simulink model "AAIver2"  (R2022a)
settings: Solver=FixedStepAuto  StartTime=0.0  StopTime=10.0  FixedStep=1e-3  RelTol=1e-3  EnableMultiTasking=on
undefined symbols (not defined in the file): D0, D10, D11, D13, D2, D3, D4, D5, D8, D9, PTA0, PTA1, PTA2, PTB23, PTB9, PTC16, PTC4, PTD0, PTD1, PTD2
libraries: frdmk64flib x10
settings Model: ExtModeTrigDuration=5  Creator=bmile  LastModifiedBy=Motz
settings OptimizationCC: EnhancedBackFolding=on  PassReuseOutputArgsAs=Individual arguments  ZeroExternalMemoryAtStartup=off  ZeroInternalMemoryAtStartup=off  MaxStackSize=64  OptimizeBlockOrder=speed  DifferentSizesBufferReuse=on  OptimizationCustomize=off  EfficientTunableParamExpr=on
settings DebuggingCC: ParameterTunabilityLossMsg=error
settings HardwareCC: ProdBitPerPointer=32  ProdBitPerSizeT=32  ProdBitPerPtrDiffT=32  ProdLargestAtomicInteger=Long  ProdLargestAtomicFloat=Double  ProdWordSize=32  ProdHWDeviceType=ARM Compatible->ARM Cortex
settings SFSimCC: MATLABDynamicMemAlloc=off
settings RTWCC: SystemTargetFile=ert.tlc  HardwareBoard=NXP FRDM-K64F  TLCOptions="-aInlineSetEventsForThisBaseRateFcn=TLC_FALSE -aSuppressMultiTaskScheduler=TLC_FALSE  -aRateBasedStepFcn=0"  TemplateMakefile=ert_default_tmf  Toolchain=GNU Tools for ARM Embedded Processors
settings CodeAppCC: ForceParamTrailComments=on  IgnoreCustomStorageClasses=off  OperatorAnnotations=on  SimulinkDataObjDesc=on  SFDataObjDesc=on  InsertBlockDesc=on
settings ERTTargetCC: ExtModeTransport=4  ExtModeMexFile=sendToCommService

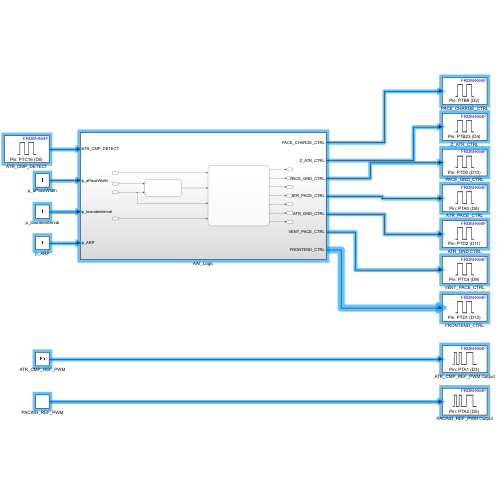
[thumbnail: Simulink's stored preview of the top-level diagram]
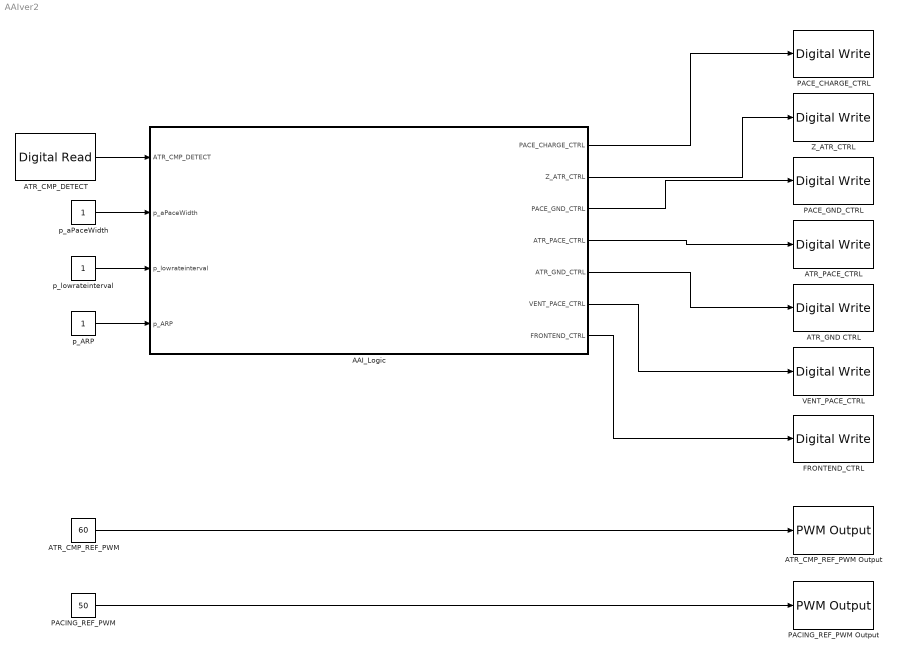
== system AAIver2 ==
  AAI_Logic : Subsystem
  ATR_CMP_DETECT : frdmk64flib/Digital Read  Whichpin=PTC16 (D0)  SampleTime=-1
  ATR_CMP_REF_PWM : Constant  Value=60
  ATR_CMP_REF_PWM Output : frdmk64flib/PWM Output  Whichpin=PTA1 (D3)  InitialFrequency=2000  InitialDutyCycle=0
  ATR_GND CTRL : frdmk64flib/Digital Write  Whichpin=PTD2 (D11)
  ATR_PACE_CTRL : frdmk64flib/Digital Write  Whichpin=PTA0 (D8)
  FRONTEND_CTRL : frdmk64flib/Digital Write  Whichpin=PTD1 (D13)
  PACE_CHARGE_CTRL : frdmk64flib/Digital Write  Whichpin=PTB9 (D2)
  PACE_GND_CTRL : frdmk64flib/Digital Write  Whichpin=PTD0 (D10)
  PACING_REF_PWM : Constant  Value=50
  PACING_REF_PWM Output : frdmk64flib/PWM Output  Whichpin=PTA2 (D5)  InitialFrequency=2000  InitialDutyCycle=0
  VENT_PACE_CTRL : frdmk64flib/Digital Write  Whichpin=PTC4 (D9)
  Z_ATR_CTRL : frdmk64flib/Digital Write  Whichpin=PTB23 (D4)
  p_ARP : Constant
  p_aPaceWidth : Constant
  p_lowrateinterval : Constant
  wires:
  PACING_REF_PWM/1 -> PACING_REF_PWM Output/1
  AAI_Logic/3(PACE_GND_CTRL) -> PACE_GND_CTRL/1
  AAI_Logic/2(Z_ATR_CTRL) -> Z_ATR_CTRL/1
  AAI_Logic/5(ATR_GND_CTRL) -> ATR_GND CTRL/1
  AAI_Logic/4(ATR_PACE_CTRL) -> ATR_PACE_CTRL/1
  p_ARP/1 -> AAI_Logic/4(p_ARP)
  p_lowrateinterval/1 -> AAI_Logic/3(p_lowrateinterval)
  AAI_Logic/6(VENT_PACE_CTRL) -> VENT_PACE_CTRL/1
  ATR_CMP_DETECT/1 -> AAI_Logic/1(ATR_CMP_DETECT)
  p_aPaceWidth/1 -> AAI_Logic/2(p_aPaceWidth)
  ATR_CMP_REF_PWM/1 -> ATR_CMP_REF_PWM Output/1
  AAI_Logic/1(PACE_CHARGE_CTRL) -> PACE_CHARGE_CTRL/1
  AAI_Logic/7(FRONTEND_CTRL) -> FRONTEND_CTRL/1

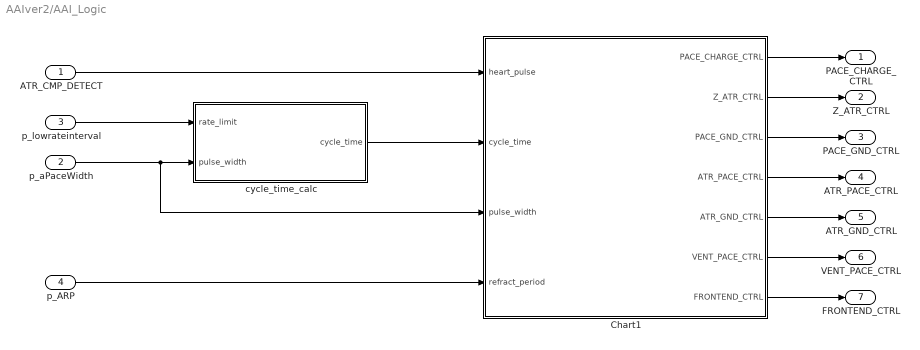
== system AAIver2/AAI_Logic ==
  ATR_CMP_DETECT : Inport
  p_aPaceWidth : Inport  Port=2
  p_lowrateinterval : Inport  Port=3
  p_ARP : Inport  Port=4
  Chart1 : Stateflow chart  TreatAsAtomicUnit=on
  cycle_time_calc : Stateflow chart  TreatAsAtomicUnit=on
  PACE_CHARGE_CTRL : Outport
  Z_ATR_CTRL : Outport  Port=2
  PACE_GND_CTRL : Outport  Port=3
  ATR_PACE_CTRL : Outport  Port=4
  ATR_GND_CTRL : Outport  Port=5
  VENT_PACE_CTRL : Outport  Port=6
  FRONTEND_CTRL : Outport  Port=7
  wires:
  cycle_time_calc/1(cycle_time) -> Chart1/2(cycle_time)
  Chart1/7(FRONTEND_CTRL) -> FRONTEND_CTRL/1
  Chart1/6(VENT_PACE_CTRL) -> VENT_PACE_CTRL/1
  Chart1/5(ATR_GND_CTRL) -> ATR_GND_CTRL/1
  Chart1/4(ATR_PACE_CTRL) -> ATR_PACE_CTRL/1
  Chart1/3(PACE_GND_CTRL) -> PACE_GND_CTRL/1
  Chart1/2(Z_ATR_CTRL) -> Z_ATR_CTRL/1
  Chart1/1(PACE_CHARGE_CTRL) -> PACE_CHARGE_CTRL/1
  p_ARP/1 -> Chart1/4(refract_period)
  p_aPaceWidth/1 -> Chart1/3(pulse_width), cycle_time_calc/2(pulse_width)
  p_lowrateinterval/1 -> cycle_time_calc/1(rate_limit)
  ATR_CMP_DETECT/1 -> Chart1/1(heart_pulse)

== stateflow chart AAIver2/AAI_Logic/cycle_time_calc ==
  state Calc_time
    entry:
    cycle_time=((1/rate_limit)*60000)-pulse_width
  (default) -> (junction 19)
  (junction 19) -> Calc_time
  data: rate_limit input; cycle_time output; pulse_width input

== stateflow chart AAIver2/AAI_Logic/Chart1 ==
  state Pulse_Sensed
    entry:
    FRONTEND_CTRL=false
  state Charging_Discharging
    entry:
    ATR_PACE_CTRL = false
    VENT_PACE_CTRL=false
    PACE_CHARGE_CTRL = true
    ATR_GND_CTRL = true
    PACE_GND_CTRL = true
    Z_ATR_CTRL=false
    FRONTEND_CTRL=true
  state Pace_Heart
    entry:
    ATR_PACE_CTRL = true
    PACE_CHARGE_CTRL = false
    PACE_GND_CTRL = true
    ATR_GND_CTRL = false
  Pulse_Sensed -> Charging_Discharging : after(refract_period,msec)
  (junction 34) -> Pulse_Sensed [order 2]
  (default) -> Charging_Discharging
  Charging_Discharging -> (junction 34)
  (junction 34) -> Pace_Heart [order 1] : [heart_pulse==true&&after(cycle_time,msec)]
  Pace_Heart -> Charging_Discharging : after(pulse_width,msec)
  data: heart_pulse input boolean; cycle_time input; PACE_CHARGE_CTRL output boolean; Z_ATR_CTRL output boolean; PACE_GND_CTRL output boolean; ATR_PACE_CTRL output boolean; ATR_GND_CTRL output boolean; pulse_width input; VENT_PACE_CTRL output boolean; refract_period input; FRONTEND_CTRL output boolean
